simulink model "psbmutual"  (Simulink 6.0)
settings: Solver=ode45  SolverMode=SingleTasking  StartTime=0.0  StopTime=0.1  RelTol=1e-3  AbsTol=1e-6
InitFcn:
  | powericon('psbinitsys',bdroot);
libraries: powerlib2 x11
settings Model: Creator=patrice  LastModifiedBy=batserve  ExtModeTrigMode=oneshot  ExtModeArmWhenConnect=off  ExtModeAutoUpdateStatusClock=off
settings DataIOCC: LimitDataPoints=off  SignalLoggingName=sigsOut
settings OptimizationCC: BlockReduction=off  BooleanDataType=off
settings DebuggingCC: SolverPrmCheckMsg=none
settings HardwareCC: TargetUnknown=on
settings RTWCC: TemplateMakefile=grt_unix.tmf

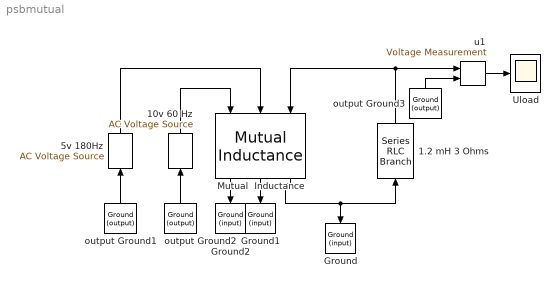
== system psbmutual ==
  1.2 mH 3 Ohms : powerlib2/Elements/Series RLC Branch  Tag=PoWeRsYsTeMbLoCk  Orientation=up  a=3  b=1.2e-03  c=inf  mesure=None  PSBOutputType=1
  10v 60 Hz : powerlib2/Electrical Sources/AC Voltage Source  Tag=PoWeRsYsTeMbLoCk  Orientation=up  A=10  P=0  F=60  stime=0  mesure=None  PSBOutputType=1
  5v 180Hz : powerlib2/Electrical Sources/AC Voltage Source  Tag=PoWeRsYsTeMbLoCk  Orientation=up  A=5  P=0  F=180  stime=0  mesure=None  PSBOutputType=1
  Ground : powerlib2/Connectors/Ground (input)  Tag=PoWeRsYsTeMbLoCk  Orientation=down
  Ground1 : powerlib2/Connectors/Ground (input)  Tag=PoWeRsYsTeMbLoCk  Orientation=down
  Ground2 : powerlib2/Connectors/Ground (input)  Tag=PoWeRsYsTeMbLoCk  Orientation=down
  Mutual  Inductance : powerlib2/Elements/Mutual Inductance  Tag=PoWeRsYsTeMbLoCk  Orientation=down  a=[1.1 1.1e-03]  b=[ 1.1 1.1e-03]  w3check=on  c=[ 1.1 1.1e-03]  d=[1.0 1.0e-03]  mesure=None  PSBOutputType=111
  Uload : Scope
      settings: TickLabels=on  TimeRange=0.1  YMin=-10  YMax=10  DataFormat=Array
  output Ground1 : powerlib2/Connectors/Ground (output)  Tag=PoWeRsYsTeMbLoCk  Orientation=up  PSBOutputType=1
  output Ground2 : powerlib2/Connectors/Ground (output)  Tag=PoWeRsYsTeMbLoCk  Orientation=up  PSBOutputType=1
  output Ground3 : powerlib2/Connectors/Ground (output)  Tag=PoWeRsYsTeMbLoCk  Orientation=up  PSBOutputType=1
  u1 : powerlib2/Measurements/Voltage Measurement  Tag=PoWeRsYsTeMmEaSuReMeNt  PhasorSimulation=off  OutputType=Magnitude  PSBOutputType=0  PSBequivalent=0
  wires:
  Mutual  Inductance/3 -> Ground/1, 1.2 mH 3 Ohms/1
  1.2 mH 3 Ohms/1 -> u1/1, Mutual  Inductance/3
  u1/1 -> Uload/1
  output Ground3/1 -> u1/2
  10v 60 Hz/1 -> Mutual  Inductance/1
  Mutual  Inductance/2 -> Ground1/1
  Mutual  Inductance/1 -> Ground2/1
  5v 180Hz/1 -> Mutual  Inductance/2
  output Ground2/1 -> 10v 60 Hz/1
  output Ground1/1 -> 5v 180Hz/1
